simulink model "momentumBasedFlight"  (R2022a)
settings: Solver=FixedStepDiscrete  StartTime=0.0  StopTime=Config.simulationTime  FixedStep=Config.tStep  RelTol=1e-3
InitFcn:
  | cd(fileparts(which(bdroot)));
  | initMomentumBasedFlight;
StopFcn:
  | cd(fileparts(which(bdroot)));
  | stopMomentumBasedFlight;
undefined symbols (not defined in the file or in its folder): biasVectorConstraint_feet, Config, ConstraintMatrix_feet, DiscIntNeverNeededParam, Frames
libraries: WBToolboxLibrary x38, momentum_flight_control_v1 x3, thrust_estimation_v1 x1, jets_control_v1 x1
(part 3 of 3)

== matlab function momentumBasedFlight/FLIGHT CONTROLLER (CORE) V3.0/Flight State Machine/Compute Gains And References/Compute Gains/Diagonalize4 ==
  data: k input; K output
function K = diagonalMatrixFromVectorFCN(k)

    K = wbc.diagonalMatrixFromVector(k);
end

== matlab function momentumBasedFlight/FLIGHT CONTROLLER (CORE) V3.0/UpdateGuiData/Update Data for the GUI ==
  data: time input
function updateVisualGuiFCN(time)

    coder.extrinsic('updateVisualGui')

    persistent updateTime

    % for now I hard-coded 0.25 [s] as updating time for the data GUI
    timeStepGui    = 0.25;

    if isempty(updateTime)
    
        updateTime = timeStepGui;
    end
    
    % update data GUI
    if time > updateTime
    
        updateVisualGui;
        updateTime = time + timeStepGui;  
    end
end

== matlab function momentumBasedFlight/FLIGHT CONTROLLER (CORE) V3.0/Flight Controller RAL-HUMANOIDS V3.0/Momentum Control for Flying/QP Solver and Integrate Contact Forces Derivative/Integrate the Contact Forces Derivative/deadZone/Deadzone Function ==
  data: u input; y output; thr input
function y = deadZoneFCN(u, thr)

    y = wbc.deadZone(u, thr);
end

== matlab function momentumBasedFlight/FLIGHT CONTROLLER (CORE) V3.0/Flight State Machine/Take Off//Landing And Fault State Detector/Vertical Forces Control ==
  data: joyButtons input; decreaseMaxFootVerticalForce output; increaseMinFootVerticalForce output; activateEqConstrTorqueControl output
function [decreaseMaxFootVerticalForce, increaseMinFootVerticalForce, activateEqConstrTorqueControl] = verticalForcesControlFCN(joyButtons)

    [decreaseMaxFootVerticalForce, increaseMinFootVerticalForce, activateEqConstrTorqueControl] = iRonCubLib_v1.verticalForcesControl(joyButtons);
end

== matlab function momentumBasedFlight/FLIGHT CONTROLLER (CORE) V3.0/Flight State Machine/Take Off//Landing And Fault State Detector/Failure Detection/MATLAB Function1 ==
  data: jetsIntensities input; rpm output; Config parameter
function rpm = thrustToRPM(jetsIntensities, Config)

    rpm = T_to_rpm(jetsIntensities, Config);

end

== matlab function momentumBasedFlight/FLIGHT CONTROLLER (CORE) V3.0/JoyStick-flightGUI Commands/Replace Joystick with Native GUI ==
  data: gui_input input; joyButtons output; joyAxes output
function [joyButtons,joyAxes] = fromGuiToJoystickFCN(gui_input)

    [joyButtons,joyAxes] = iRonCubLib_v1.fromGuiToJoystick(gui_input);
end

== matlab function momentumBasedFlight/FLIGHT CONTROLLER (CORE) V3.0/JoyStick-flightGUI Commands/Autopilot ==
  data: time input; joyButtons output; joyAxes output
function [joyButtons,joyAxes] = autopilotFCN(time)

    [joyButtons,joyAxes] = autopilotFCN(time);
end

== matlab function momentumBasedFlight/FLIGHT CONTROLLER (CORE) V3.0/Flight Controller RAL-HUMANOIDS V3.0/Momentum Control for Flying/QP Solver and Integrate Contact Forces Derivative/Integrate the Contact Forces Derivative/Select Integrator Initial Condition ==
  data: feetContactIsActive input; contactForces input; contactForces_0 output
function contactForces_0 = selectInitContactForcesFCN(feetContactIsActive, contactForces)

    contactForces_0 = iRonCubLib_v1.selectInitContactForces(feetContactIsActive, contactForces);
end

== matlab function momentumBasedFlight/FLIGHT CONTROLLER (CORE) V3.0/Flight State Machine/Compute Gains And References/Trajectory Generator/Compute CoM and Base Rotation References ==
  data: posCoM_init input; w_R_b_init input; jointPos_init input; moveFront input; pos_vel_acc_jerk_CoM_des output; moveLateral input; moveUpDown input; rotateRoll input; rotatePitch input; rotateYaw input; turbo_mode input; goLandingPos input; feetContactIsActive input; oneFootIsInContact input; turbinesStatus input; t input; Config parameter; rot_vel_acc_jerk_base_des output; jointPos_des output
function [pos_vel_acc_jerk_CoM_des, rot_vel_acc_jerk_base_des, jointPos_des] = ...
             computeReferencesBaseAndCoMFCN(posCoM_init, w_R_b_init,jointPos_init, moveFront, moveLateral, moveUpDown, rotateRoll, rotatePitch, ...
                                            rotateYaw, turbo_mode, goLandingPos, feetContactIsActive, oneFootIsInContact, turbinesStatus, t, Config)
                                     
    [pos_vel_acc_jerk_CoM_des, rot_vel_acc_jerk_base_des, jointPos_des] = ...
        computeReferencesBaseAndCoM(posCoM_init, w_R_b_init, jointPos_init,moveFront, moveLateral, moveUpDown, rotateRoll, rotatePitch, ...
                                    rotateYaw, turbo_mode, goLandingPos, feetContactIsActive, oneFootIsInContact, turbinesStatus, t, Config);
end

== matlab function momentumBasedFlight/FLIGHT CONTROLLER (CORE) V3.0/Flight State Machine/Compute Gains And References/Trajectory Generator/Detect Robot Movement Request From Joystick ==
  data: joyAxes input; moveFront output; moveLateral output; moveUpDown output; rotateRoll output; rotatePitch output; joyButtons input; rotateYaw output; turbo_mode output; goLandingPos output
function [moveFront,moveLateral,moveUpDown,rotateRoll,rotatePitch,rotateYaw,turbo_mode,goLandingPos] = detectMovementsFromJoystickFCN(joyAxes,joyButtons)

    [moveFront,moveLateral,moveUpDown,rotateRoll,rotatePitch,rotateYaw,turbo_mode,goLandingPos] = iRonCubLib_v1.detectMovementsFromJoystick(joyAxes,joyButtons);
end

== matlab function momentumBasedFlight/FLIGHT CONTROLLER (CORE) V3.0/Flight State Machine/Compute Gains And References/Smooth CoM and Base References/Smooth Reference Orientations/Rotational PID Controller/Compute Rotation Matrix Derivative ==
  data: gainSmoothingBaseRot input; w_R_b_des input; w_R_b input; b_omega_b output; RDot output
function [b_omega_b, RDot] = rotationDerivativeFromAngVelFCN(gainSmoothingBaseRot, w_R_b_des, w_R_b)
                                                                                                                                                            
    % Rotational PID: 
    %
    % w_R_b_des = reference rotation (may be discontinuous)
    % 
    % b_omega_b = control input for the rotational PID. The angular velocity
    %             is expressed w.r.t. a frame attached to the link, i.e. it 
    %             is expressed in the "body" frame (b).
    % 
    % Kp        = control gain
    %
    % w_R_b     = smooth base rotation
    %
    b_omega_b_des       = zeros(3,1);
    Kp                  = gainSmoothingBaseRot;
    b_omega_b           = wbc.rotationalPID_bodyVelocity(w_R_b, w_R_b_des, b_omega_b_des, Kp);
                      
    % compute the rotation matrix derivative given the angular velocity in body frame
    RDot                = wbc.rotationDerivativeFromBodyAngVel(b_omega_b, w_R_b); 
end

== matlab function momentumBasedFlight/Visualizer/Task and Base Frame Kinematics/MATLAB Function1 ==
  data: RPY_Corr output; rollPitchYaw input
function RPY_Corr = correctYawAngleFCN(rollPitchYaw)

    RPY_Corr = correctYawAngle(rollPitchYaw);

end

== matlab function momentumBasedFlight/FLIGHT CONTROLLER (CORE) V3.0/Flight Controller RAL-HUMANOIDS V3.0/Joint Torque Control for Flying/QP torqueControl/Process QP Inputs Torque Control ==
  data: HessianMatrixQP input; H_balancing output; gVectorQP input; InequalityConstrMatrix input; biasVectorInequalityConstr input; g_balancing output; ub_balancing output; lb_balancing output; Aeq_balancing output; lbEq_balancing output; ubEq_balancing output; H_flight output; g_flight output; ub_flight output; lb_flight output; jointTorquesSaturation input; Config parameter
function [H_balancing,g_balancing,ub_balancing,lb_balancing,Aeq_balancing,lbEq_balancing,ubEq_balancing, ...
          H_flight,g_flight,ub_flight,lb_flight] = processQPinputTorqueControlFCN ...
                                                       (HessianMatrixQP,gVectorQP,InequalityConstrMatrix, ...
                                                        biasVectorInequalityConstr,jointTorquesSaturation,Config)   
   
[H_balancing,g_balancing,ub_balancing,lb_balancing,Aeq_balancing,lbEq_balancing,ubEq_balancing, ...
          H_flight,g_flight,ub_flight,lb_flight] = iRonCubLib_v1.processQPinputTorqueControl ...
                                                       (HessianMatrixQP,gVectorQP,InequalityConstrMatrix, ...
                                                        biasVectorInequalityConstr,jointTorquesSaturation,Config);     
end
